simulink model "ff_regulator"  (R2022b)
settings: Solver=ode23t  StartTime=0.0  StopTime=19.7  RelTol=1e-3  EnableMultiTasking=on
undefined symbols (not defined in the file): ff_Kd, ff_Kp, hp6
libraries: roblocks x5
settings Model: Creator=corkep  LastModifiedBy=sam
settings SolverCC: AlgebraicLoopSolver=TrustRegion
settings DataIOCC: LimitDataPoints=on  SaveFormat=Array  SignalLoggingSaveFormat=ModelDataLogs  TimeSaveName=t  OutputSaveName=y  ReturnWorkspaceOutputsName=fforward
settings OptimizationCC: ExpressionDepthLimit=2147483647  LifeSpan=inf
settings DebuggingCC: UnderspecifiedInitializationDetection=Classic  MergeDetectMultiDrivingBlocksExec=none  SolverPrmCheckMsg=warning  FcnCallInpInsideContextMsg=warning  UnconnectedInputMsg=warning  UnconnectedOutputMsg=warning  UnconnectedLineMsg=warning  AllowSymbolicDim=off  StateNameClashWarn=warning  SFUnexpectedBacktrackingDiag=warning  SFNoUnconditionalDefaultTransitionDiag=warning  SFExecutionAtInitializationDiag=none  SFMachineParentedDataDiag=warning  ArithmeticOperatorsInVariantConditions=warning
settings HardwareCC: ProdBitPerPointer=32  ProdBitPerSizeT=32  ProdBitPerPtrDiffT=32  ProdLargestAtomicFloat=None  ProdIntDivRoundTo=Undefined  ProdEndianess=Unspecified  ProdWordSize=32  ProdHWDeviceType=32-bit Generic
settings ModelReferenceCC: EnableRefExpFcnMdlSchedulingChecks=on  PropagateSignalLabelsOutOfModel=off
settings SFSimCC: SimUseLocalCustomCode=off  CustomCodeUndefinedFunction=UseInterfaceOnly
settings RTWCC: RTWUseLocalCustomCode=off
settings CodeAppCC: StateflowObjectComments=on
settings GRTTargetCC: TargetLangStandard=C89/C90 (ANSI)  CombineOutputUpdateFcns=off  GRTInterface=on
settings ConfigComp: CovMetricSettings=dw  CovSaveCumulativeToWorkspaceVar=on  CovSaveSingleToWorkspaceVar=on  CovExternalEMLEnable=off

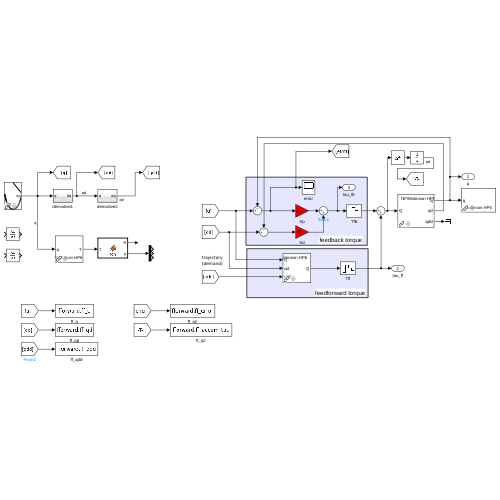
[thumbnail: Simulink's stored preview of the top-level diagram]
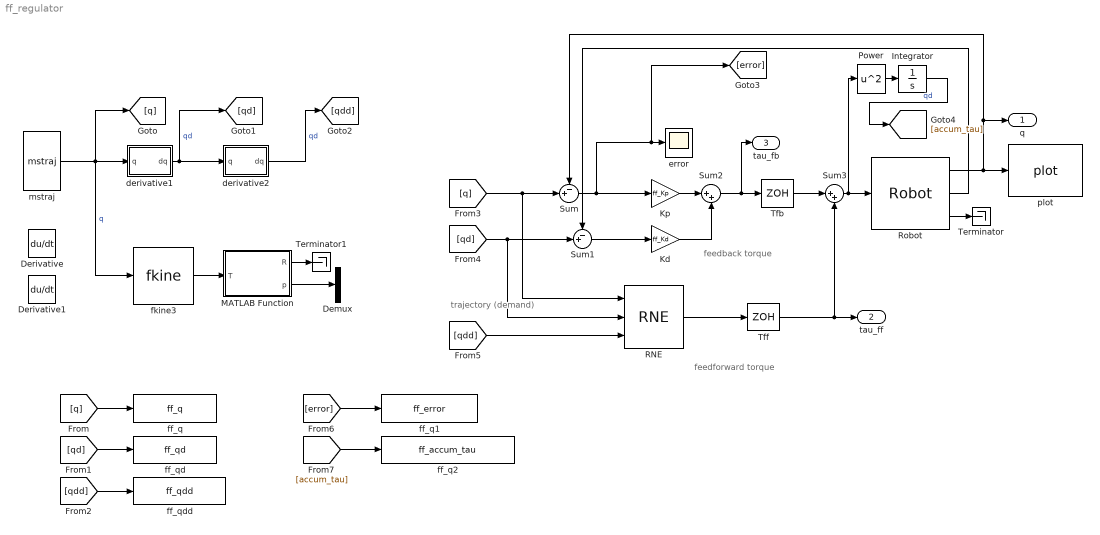
== system ff_regulator ==
  note: feedback torque
  note: trajectory
      | (demand)
  note: feedforward torque
  Demux : Demux  Outputs=3
  Derivative : Derivative
  Derivative1 : Derivative
  Integrator : Integrator
  Kd : Gain  Gain=ff_Kd  SaturateOnIntegerOverflow=on  OutDataTypeStr=Inherit: Same as input  ParamDataTypeStr=Inherit: Same as input
  Kp : Gain  Gain=ff_Kp  SaturateOnIntegerOverflow=on  OutDataTypeStr=Inherit: Same as input  ParamDataTypeStr=Inherit: Same as input
  MATLAB Function : MATLAB Function  TreatAsAtomicUnit=on
  Power : Math  Operator=square
  RNE : roblocks/Arm/RNE  robot=hp6.nofriction()  grav=[0 0 9.81]
  Robot : roblocks/Arm/Robot  robot=hp6.nofriction  q0=[0 0 0 0 0 0]
  Sum : Sum  Inputs=-+|  InputSameDT=on  SaturateOnIntegerOverflow=on  OutDataTypeStr=Inherit: Same as first input
  Sum1 : Sum  Inputs=-+|  InputSameDT=on  SaturateOnIntegerOverflow=on  OutDataTypeStr=Inherit: Same as first input
  Sum2 : Sum  Inputs=|++  InputSameDT=on  SaturateOnIntegerOverflow=on  OutDataTypeStr=Inherit: Same as first input
  Sum3 : Sum  Inputs=|++  InputSameDT=on  SaturateOnIntegerOverflow=on  OutDataTypeStr=Inherit: Same as first input
  Terminator : Terminator
  Terminator1 : Terminator
  Tfb : ZeroOrderHold  SampleTime=0.002
  Tff : ZeroOrderHold  SampleTime=0.05
  derivative1 : Subsystem
  derivative2 : Subsystem
  error : Scope
  ff_q : ToWorkspace  VariableName=ff_q  SaveFormat=Timeseries  SampleTime=-1
  ff_q1 : ToWorkspace  VariableName=ff_error  SaveFormat=Timeseries  SampleTime=-1
  ff_q2 : ToWorkspace  VariableName=ff_accum_tau  SaveFormat=Timeseries  SampleTime=-1
  ff_qd : ToWorkspace  VariableName=ff_qd  SaveFormat=Timeseries  SampleTime=-1
  ff_qdd : ToWorkspace  VariableName=ff_qdd  SaveFormat=Timeseries  SampleTime=-1
  fkine3 : roblocks/Arm/fkine  robot=hp6
  mstraj : roblocks/Toolbox/mstraj  path=pathFull2  vaxis=[2 2 2 2 2 2]  tseg=[]  dt=0.1  tacc=0.3  setsimtime=on
  plot : roblocks/Arm/plot  robot=hp6  fps=10  holdplot=on
  q : Outport
  tau_ff : Outport  Port=2
  tau_fb : Outport  Port=3
  wires:
  Kd/1 -> Sum2/2
  Sum/1 -> [error], error/1, Kp/1
  Kp/1 -> Sum2/1
  Sum1/1 -> Kd/1
  Sum2/1 -> Tfb/1, tau_fb/1
  Sum3/1 -> Power/1, Robot/1
  Robot/1 -> Sum/1, q/1, plot/1
  Robot/2 -> Sum1/1
  Robot/3 -> Terminator/1
  RNE/1 -> Tff/1
  Tff/1 -> Sum3/2, tau_ff/1
  Tfb/1 -> Sum3/1
  mstraj/1 -> derivative1/1(q), fkine3/1, [q]  "q"
  fkine3/1 -> MATLAB Function/1(T)
  MATLAB Function/2(p) -> Demux/1
  MATLAB Function/1(R) -> Terminator1/1
  derivative1/1(dq) -> derivative2/1(q), [qd]  "qd"
  [qdd] -> ff_qdd/1
  [qd] -> ff_qd/1
  [q] -> ff_q/1
  derivative2/1(dq) -> [qdd]  "qd"
  [qd] -> RNE/2, Sum1/2
  [qdd] -> RNE/3
  [q] -> RNE/1, Sum/2
  Power/1 -> Integrator/1
  Integrator/1 -> [accum_tau]  "qd"
  [error] -> ff_q1/1
  [accum_tau] -> ff_q2/1

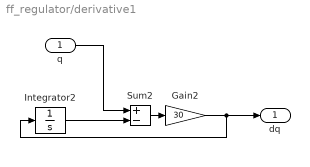
== system ff_regulator/derivative1 ==
  q : Inport
  Gain2 : Gain  Gain=30
  Integrator2 : Integrator
  Sum2 : Sum  Inputs=+-
  dq : Outport
  wires:
  q/1 -> Sum2/1
  Integrator2/1 -> Sum2/2
  Sum2/1 -> Gain2/1
  Gain2/1 -> dq/1, Integrator2/1

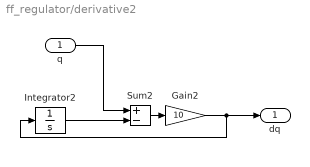
== system ff_regulator/derivative2 ==
  q : Inport
  Gain2 : Gain  Gain=10
  Integrator2 : Integrator
  Sum2 : Sum  Inputs=+-
  dq : Outport
  wires:
  q/1 -> Sum2/1
  Integrator2/1 -> Sum2/2
  Sum2/1 -> Gain2/1
  Gain2/1 -> dq/1, Integrator2/1

== matlab function ff_regulator/MATLAB Function ==
  data: T input; R output; p output
function [R, p] = fcn(T)

p = T([1,2,3],4);
R = T([1,2,3],[1,2,3]);
